simulink model "simple"  (R2012b)
settings: Solver=ode45  StartTime=0.0  StopTime=10.0  RelTol=1e-3
settings Model: Creator=ana  LastModifiedBy=ana

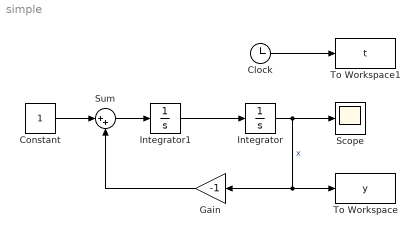
== system simple ==
  Clock : Clock
  Constant : Constant
  Gain : Gain  Gain=-1
  Integrator : Integrator  InitialCondition=5
  Integrator1 : Integrator
  Scope : Scope
  Sum : Sum  Inputs=|++
  To Workspace : ToWorkspace  VariableName=y  SampleTime=-1
  To Workspace1 : ToWorkspace  VariableName=t  SampleTime=-1
  wires:
  Integrator/1 -> Scope/1, Gain/1, To Workspace/1  "x"
  Integrator1/1 -> Integrator/1
  Sum/1 -> Integrator1/1
  Gain/1 -> Sum/2
  Constant/1 -> Sum/1
  Clock/1 -> To Workspace1/1
